simulink library "uavsimBlocksetLinearAerodynamicCoefficient"  (Simulink 8.0)
settings: Solver=ode45  StartTime=0.0  StopTime=10.0  RelTol=1e-3
settings Model: Creator=mstolle  LastModifiedBy=j.bolting

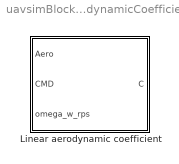
== system uavsimBlocksetLinearAerodynamicCoefficient ==
  Linear aerodynamic coefficient : Subsystem  mask{mask_C_0=0, mask_C_alpha=0, mask_C_beta=0, mask_C_alphaDot=0, mask_C_betaDot=0, mask_C_p=0, mask_C_q=0, mask_C_r=0, mask_C_delta_a=0, mask_C_delta_e=0, mask_C_delta_r=0, mask_C_delta_f=0, mask_C_Mach=0}
      mask prompts: mask_C_0 "C_0"; mask_C_alpha "C_alpha"; mask_C_beta "C_beta"; mask_C_alphaDot "C_alphaDot"; mask_C_betaDot "C_betaDot"; mask_C_p "C_p"; mask_C_q "C_q"; mask_C_r "C_r"; mask_C_delta_a "C_delta_a"; mask_C_delta_e "C_delta_e"; mask_C_delta_r "C_delta_r"; mask_C_delta_f "C_delta_f"; mask_C_Mach "C_Mach"

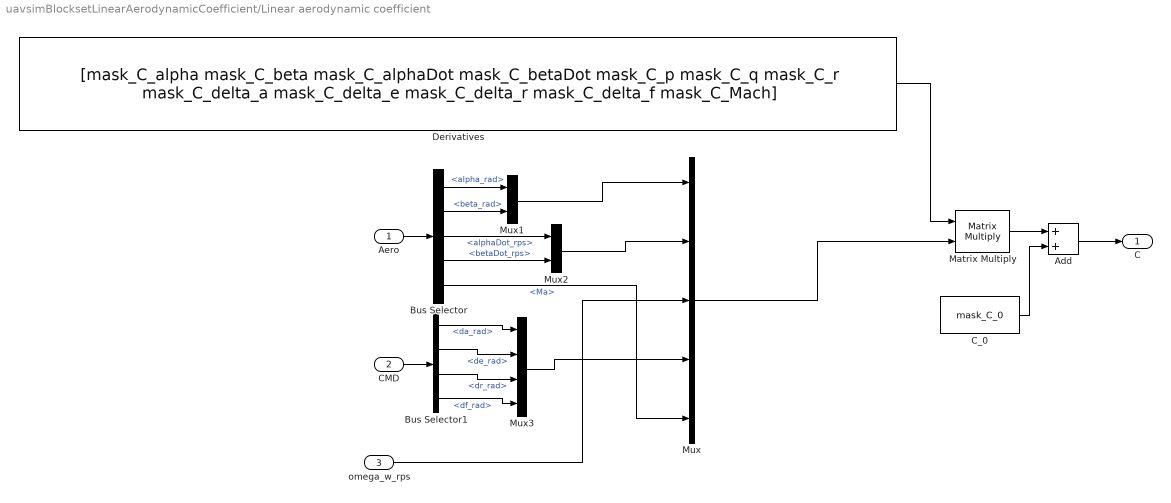
== system uavsimBlocksetLinearAerodynamicCoefficient/Linear aerodynamic coefficient ==
  Aero : Inport  OutDataTypeStr=Bus: Aero
  CMD : Inport  Port=2  OutDataTypeStr=Bus: CMD
  omega_w_rps : Inport  Port=3
  Add : Sum
  Bus Selector : BusSelector  OutputSignals=alpha_rad,beta_rad,alphaDot_rps,betaDot_rps,Ma
  Bus Selector1 : BusSelector  OutputSignals=da_rad,de_rad,dr_rad,df_rad
  C_0 : Constant  Value=mask_C_0
  Derivatives : Constant  Value=[mask_C_alpha mask_C_beta mask_C_alphaDot mask_C_betaDot mask_C_p mask_C_q mask_C_r mask_C_delta_a mask_C_delta_e mask_C_delta_r mask_C_delta_f mask_C_Mach]  VectorParams1D=off
  Matrix Multiply : Product  Multiplication=Matrix(*)
  Mux : Mux  Inputs=5
  Mux1 : Mux  Inputs=2
  Mux2 : Mux  Inputs=2
  Mux3 : Mux
  C : Outport
  wires:
  Mux1/1 -> Mux/1
  Mux/1 -> Matrix Multiply/2
  Derivatives/1 -> Matrix Multiply/1
  omega_w_rps/1 -> Mux/3
  Bus Selector/5 -> Mux/5  "<Ma>"
  Add/1 -> C/1
  Matrix Multiply/1 -> Add/1
  C_0/1 -> Add/2
  Mux2/1 -> Mux/2
  Aero/1 -> Bus Selector/1
  Bus Selector/1 -> Mux1/1  "<alpha_rad>"
  Bus Selector/2 -> Mux1/2  "<beta_rad>"
  Bus Selector/3 -> Mux2/1  "<alphaDot_rps>"
  Bus Selector/4 -> Mux2/2  "<betaDot_rps>"
  CMD/1 -> Bus Selector1/1
  Bus Selector1/1 -> Mux3/1  "<da_rad>"
  Bus Selector1/2 -> Mux3/2  "<de_rad>"
  Bus Selector1/3 -> Mux3/3  "<dr_rad>"
  Bus Selector1/4 -> Mux3/4  "<df_rad>"
  Mux3/1 -> Mux/4
